simulink model "Electrical_sol"  (R2018b)
settings: Solver=VariableStepAuto  StartTime=0.0  StopTime=10.0  RelTol=1e-3
values from neighbouring files (symbols this model uses):
  Jeq = Jm+Jh+Jp    (= 1.120304e-05)    [QuanserData.m]
  k1 = 1.2e-5    (= 1.2e-05)    [QuanserData.m]
  k2 = 3.54e-9    (= 3.54e-09)    [QuanserData.m]
  k3 = 0    [QuanserData.m]
  k4 = 6.23e-7    (= 6.23e-07)    [QuanserData.m]
  km = 0.042    [QuanserData.m]
  Lm = 1.16e-3    (= 0.00116)    [QuanserData.m]
  Rm = 8.4    [QuanserData.m]
settings Model: Creator=y.briere  LastModifiedBy=y.briere
settings DataIOCC: ExternalInput=[0 15]  InitialState=[]
settings OptimizationCC: DefaultParameterBehavior=Inlined  BufferReuse=off
settings DebuggingCC: InitInArrayFormatMsg=none

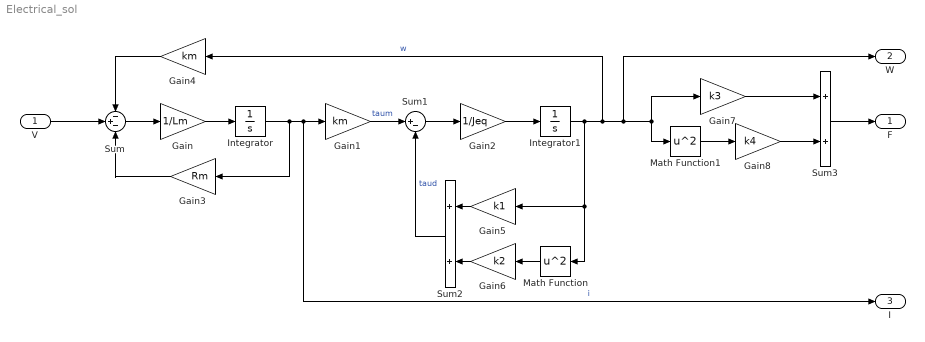
== system Electrical_sol ==
  V : Inport
  Gain : Gain  Gain=1/Lm
  Gain1 : Gain  Gain=km
  Gain2 : Gain  Gain=1/Jeq
  Gain3 : Gain  Gain=Rm
  Gain4 : Gain  Gain=km
  Gain5 : Gain  Gain=k1
  Gain6 : Gain  Gain=k2
  Gain7 : Gain  Gain=k3
  Gain8 : Gain  Gain=k4
  Integrator : Integrator
  Integrator1 : Integrator
  Math Function : Math  Operator=square  SaturateOnIntegerOverflow=on
  Math Function1 : Math  Operator=square  SaturateOnIntegerOverflow=on
  Sum : Sum  Inputs=-+-
  Sum1 : Sum  Inputs=|+-
  Sum2 : Sum
  Sum3 : Sum
  F : Outport
  W : Outport  Port=2
  I : Outport  Port=3
  wires:
  V/1 -> Sum/2
  Sum1/1 -> Gain2/1
  Sum/1 -> Gain/1
  Gain/1 -> Integrator/1
  Integrator/1 -> I/1, Gain1/1, Gain3/1  "i"
  Gain1/1 -> Sum1/1  "taum"
  Gain2/1 -> Integrator1/1
  Gain3/1 -> Sum/3
  Integrator1/1 -> Gain5/1, Math Function/1, W/1, Gain7/1, Math Function1/1, Gain4/1  "w"
  Gain4/1 -> Sum/1
  Sum2/1 -> Sum1/2  "taud"
  Gain5/1 -> Sum2/1
  Gain6/1 -> Sum2/2
  Math Function/1 -> Gain6/1
  Sum3/1 -> F/1
  Gain7/1 -> Sum3/1
  Math Function1/1 -> Gain8/1
  Gain8/1 -> Sum3/2
